simulink model "newnewPMSG"  (R2025b)
settings: Solver=VariableStepAuto  StartTime=0.0  StopTime=0.5  RelTol=1e-3
libraries: fl_lib x30, nesl_utility x19, ee_lib x8, simulink x7, slpidlib x6, eeTransforms x4, eePowerMeasurement x1, eeSinusoidalMeasurementV2 x1, mcbeeMathTransformLib x1
(part 1 of 2)
settings Model: SimulationMode=accelerator  Creator=zxd3816  LastModifiedBy=agarcian
settings SolverCC: AlgebraicLoopSolver=TrustRegion
settings DebuggingCC: UnconnectedInputMsg=warning  UnconnectedOutputMsg=warning  UnconnectedLineMsg=warning
settings ModelReferenceCC: EnableRefExpFcnMdlSchedulingChecks=on
settings RTWCC: GPUComputeCapability=3.5  DLArmComputeVersion=19.05

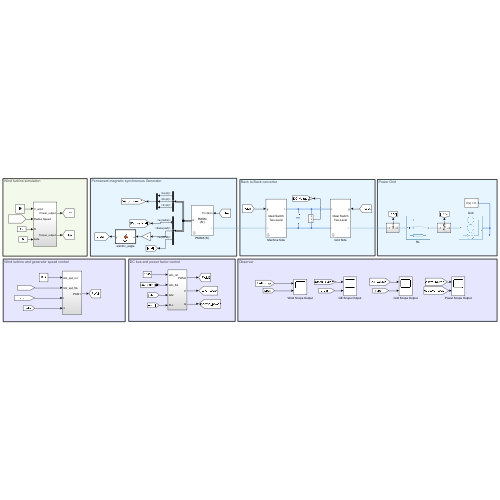
[thumbnail: Simulink's stored preview of the top-level diagram]
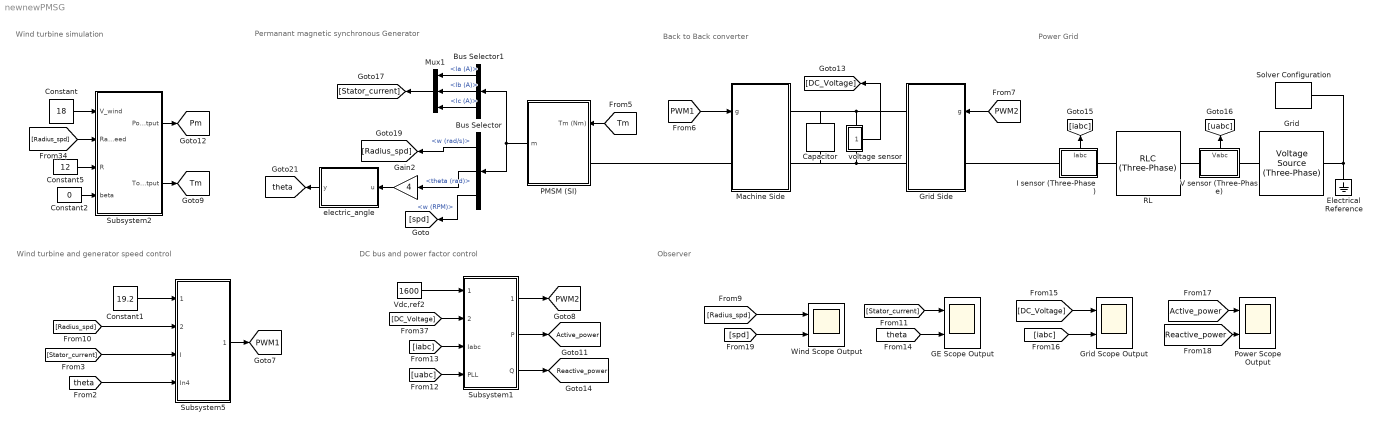
== system newnewPMSG ==
  note: DC bus and power factor control
  note: Wind turbine and generator speed control
  note: Wind turbine simulation
  note: Permanant magnetic synchronous Generator
  note: Power Grid
  note: Back to Back converter
  note: Observer
  Bus Selector : BusSelector  OutputSignals=w (rad/s),theta (rad),w (RPM)
  Bus Selector1 : BusSelector  OutputSignals=Ia (A),Ib (A),Ic (A)
  Capacitor : fl_lib/Electrical/Electrical Elements/Capacitor  c=5000e-5 F  r=0 Ohm  g=0 1/Ohm  i_specify=off  i_priority=None  i=0 A  i_nominal_specify=off  i_nominal_value=1  i_nominal_unit=A  v_specify=off  v_priority=None  v=0 V  v_nominal_specify=off  v_nominal_value=1  v_nominal_unit=V  vc_specify=on  vc_priority=High  vc=1600 V  vc_nominal_specify=off  vc_nominal_value=1  vc_nominal_unit=V
  Constant : Constant  Value=18
  Constant1 : Constant  Value=19.2
  Constant2 : Constant  Value=0
  Constant5 : Constant  Value=12
  Electrical Reference : fl_lib/Electrical/Electrical Elements/Electrical Reference
  GE Scope Output : Scope  NumInputPorts=2
      settings: ActiveDisplayYMinimum=-1886.54614  ActiveDisplayYMaximum=1887.1481  DataLoggingDecimation=10  DataLoggingVariableName=GE
  Gain2 : Gain  Gain=4
  Grid : ee_lib/Sources/Voltage Source (Three-Phase)  vline_rms=400*sqrt(3) V  shift=0 deg  freq=60 Hz  impedance_option=0  SShortCircuit=1e6 A*V  XR=15  R=0.01 Ohm  L=3.97e-4 H  harmonic_option=0  harmonic_orders=[5, 7, 11, 13]  harmonic_ratios=[.1, .1, .1, .1]  G_parasitic=0 1/Ohm  I_specify=off  I_priority=None  I=[0, 0, 0] A  I_nominal_specify=off  I_nominal_value=1  I_nominal_unit=A
  Grid Scope Output : Scope  NumInputPorts=2
      settings: ActiveDisplayYMinimum=1597.69606  ActiveDisplayYMaximum=1613.06273  DataLoggingDecimation=10  DataLoggingVariableName=Grid
  Grid Side : Subsystem  mask{Vf=1e-3, Ron=1e-3, Goff=1e-5, run_time=off}
      mask prompts: Vf "Forward Voltage (Vf)"; Ron "On Resistance (Ohm)"; Goff "Off Conductance (1/Ohm)"; run_time "Set parameters to run-time (model does not recompile if parameters change value)"
      mask Callback run_time:
      | run_time = get_param(gcb,'run_time');
      | 
      | path_converter = [gcb,'/converter'];
      | 
      | switch run_time
      |     case 'off'
      |         pcr = 'compiletime';
      |     case 'on'
      |         pcr = 'runtime';
      | end
      | 
      | set_param(path_converter,'Ron_conf',pcr)
      | set_param(path_converter,'Goff_conf',pcr)
      | set_param(path_converter,'Vf_conf',pcr)
      mask DialogControl DescGroupVar Prompt: Two-Level Converter
      mask Display: disp('Ideal Switch\nTwo-Level')
  I sensor (Three-Phase) : Subsystem
      settings: PortSchema="{\"entries\":[{\"content\":{\"sides\":[{\"content\":{\"connectorIds\":[\"LConn1\"]},\"type\":\"ConnectorPlacement.EquallySpacedRectSide\",\"uuid\":\"66880061-d275-464c-ab2c-563a1dd2cd8b\"},{\"content\":{\"connectorIds\":[\"RConn1\"],\"side\":\"RIGHT\"},\"type\":\"ConnectorPlacement.EquallySpacedRectSide\",\"uuid\":\"61b04713-3835-4ea6-b554-2bb2ace28c8c\"},{\"content\":{\"connectorIds\":[\"Out1\"],\"side\":\"TOP\"},\"type\":\"ConnectorPlacement.EquallySpacedRectSide\",\"uuid\":\"be795a7c-014c-44ea-ab59-513af0394dbb\"}]},\"type\":\"ConnectorPlacement.EquallySpacedConnector\",\"uuid\":\"739e21ea-20b0-4a9e-9950-77186c3d44aa\"}],\"packageUris\":[\"http://schema.mathworks.com/mf0/Connector/R2020b\"],\"version\":\"1.0\"}"
  Machine Side : Subsystem  mask{Vf=1e-3, Ron=1e-3, Goff=1e-5, run_time=off}
      mask prompts: Vf "Forward Voltage (Vf)"; Ron "On Resistance (Ohm)"; Goff "Off Conductance (1/Ohm)"; run_time "Set parameters to run-time (model does not recompile if parameters change value)"
      mask Callback run_time:
      | run_time = get_param(gcb,'run_time');
      | 
      | path_converter = [gcb,'/converter'];
      | 
      | switch run_time
      |     case 'off'
      |         pcr = 'compiletime';
      |     case 'on'
      |         pcr = 'runtime';
      | end
      | 
      | set_param(path_converter,'Ron_conf',pcr)
      | set_param(path_converter,'Goff_conf',pcr)
      | set_param(path_converter,'Vf_conf',pcr)
      mask DialogControl DescGroupVar Prompt: Two-Level Converter
      mask Display: disp('Ideal Switch\nTwo-Level')
  Mux1 : Mux  Inputs=3
  PMSM (SI) : Subsystem  mask{p=4, flux_linkage=1, Ld=0.001, Lq=0.001, Rs=0.005, J=0.5, D=0}
      mask prompts: p "pole pairs"; flux_linkage "Flux linkage (Wb)"; Ld "Stator d-axis inductance (H)"; Lq "Stator q-axis inductance (H)"; Rs "Stator resistance per phase (Ohm)"; J "Rotor inertia (kg*m^2)"; D "Rotor damping (N*m*s/rad)"
      mask DialogControl DescGroupVar Prompt: PMSM (SI)
      mask Display: disp('PMSM\n(SI)')
  Power Scope Output : Scope  NumInputPorts=2
      settings: ActiveDisplayYMinimum=-41950.10673  ActiveDisplayYMaximum=152400.48726  DataLoggingDecimation=10  DataLoggingVariableName=power
  RL : ee_lib/Passive/RLC Assemblies/RLC (Three-Phase)  port_option=ee.enum.threePhasePort.composite  component_structure=ee.enum.rlc.structure.SeriesRL  R=3/8 Ohm  L=3e-3 H  C=1e-6 F  R_parasitic=0 Ohm  G_parasitic=0 1/Ohm  IL_specify=off  IL_priority=High  IL=[0, 0, 0] A  IL_nominal_specify=off  IL_nominal_value=1  IL_nominal_unit=A  VC_specify=off  VC_priority=High  VC=[0, 0, 0] V  VC_nominal_specify=off  VC_nominal_value=1  VC_nominal_unit=V
      settings: InternalSimscapePortConfiguration="{\"Bottom\":[],\"Left\":[{\"id\":\"N1\",\"label\":\"~1\",\"type\":\"foundation.electrical.three_phase\"}],\"Right\":[{\"id\":\"N2\",\"label\":\"~2\",\"type\":\"foundation.electrical.three_phase\"}],\"Top\":[]}"
  Solver Configuration : nesl_utility/Solver Configuration  PhysicalDomain=network_engine_domain  SubClassName=solver  LeftPortType=input  RightPortType=generic  Tones=[]  Harmonics=[]  SimulateNoise=off  Profile=off  UseLocalSampling=off  EnableSwitchedLinearOptims=on  FrequencyDomain=off  UseCCode=off  RelTol=0.001  AbsTol=0.001  MinStep=1e-09  ToWorkspace=off  RevertToSquareIcSolve=off  NumHomotopyIterations=100  PhasorMode=off  PhasorModeNumHarmonics=1  ConsistencySolver=NEWTON_XTOL_AFTER_FTOL  IndexReductionMethod=None  DoDC=off  ResidualTolerance=1e-09  ConsistencyTolSource=GLOBAL  ConsistencyAbsTol=0.001  ConsistencyRelTol=0.001  ConsistencyTolFactor=0.001  UseLocalSolver=on  LocalSolverChoice=NE_PARTITIONING_ADVANCER  ResolveIndetEquations=off  FunctionEvalNumThread=1  LocalSolverSampleTime=5e-6  DoFixedCost=off  MaxNonlinIter=1  MaxModeIter=2  ComputeImpulses=off  ImpulseIterations=2  LinearAlgebra=auto  LinearAlgebraNumThread=0  EquationFormulation=NE_TIME_EF  DelaysMemoryBudget=1024  AutomaticFiltering=off  FilteringTimeConstant=0.001  PartitionStorageMethod=AS_NEEDED  PartitionMemoryBudget=1024  PartitionMethod=ROBUST  MultibodyUseLocalSolver=off  MultibodyLocalSolverChoice=ODE1  MultibodyLocalSolverSampleTime=0.001
  Subsystem1 : Subsystem
  Subsystem2 : Subsystem
  Subsystem5 : Subsystem
  V sensor (Three-Phase) : Subsystem
      settings: PortSchema="{\"entries\":[{\"content\":{\"sides\":[{\"content\":{\"connectorIds\":[\"LConn1\"]},\"type\":\"ConnectorPlacement.EquallySpacedRectSide\",\"uuid\":\"66880061-d275-464c-ab2c-563a1dd2cd8b\"},{\"content\":{\"connectorIds\":[\"RConn1\"],\"side\":\"RIGHT\"},\"type\":\"ConnectorPlacement.EquallySpacedRectSide\",\"uuid\":\"61b04713-3835-4ea6-b554-2bb2ace28c8c\"},{\"content\":{\"connectorIds\":[\"Out1\"],\"side\":\"TOP\"},\"type\":\"ConnectorPlacement.EquallySpacedRectSide\",\"uuid\":\"be795a7c-014c-44ea-ab59-513af0394dbb\"}]},\"type\":\"ConnectorPlacement.EquallySpacedConnector\",\"uuid\":\"739e21ea-20b0-4a9e-9950-77186c3d44aa\"}],\"packageUris\":[\"http://schema.mathworks.com/mf0/Connector/R2020b\"],\"version\":\"1.0\"}"
  Vdc,ref2 : Constant  Value=1600
  Wind Scope Output : Scope  NumInputPorts=2
      settings: ActiveDisplayYMinimum=-2.5199526294188392  ActiveDisplayYMaximum=22.679573664769556  DataLoggingDecimation=10  DataLoggingVariableName=wind
  electric_angle : MATLAB Function  TreatAsAtomicUnit=on
  voltage sensor : Subsystem
      settings: PortSchema="{\"entries\":[{\"content\":{\"sides\":[{\"content\":{},\"type\":\"ConnectorPlacement.EquallySpacedRectSide\",\"uuid\":\"799648ba-196f-427a-9565-f64fffdae700\"},{\"content\":{\"connectorIds\":[\"Out1\"],\"side\":\"RIGHT\"},\"type\":\"ConnectorPlacement.EquallySpacedRectSide\",\"uuid\":\"662de5d5-c2ef-406c-9235-94a35f9d89fb\"},{\"content\":{\"connectorIds\":[\"LConn1\"],\"side\":\"TOP\"},\"type\":\"ConnectorPlacement.EquallySpacedRectSide\",\"uuid\":\"67dc8fec-98bd-426f-bbe6-5723f2587b12\"},{\"content\":{\"connectorIds\":[\"RConn1\"],\"side\":\"BOTTOM\"},\"type\":\"ConnectorPlacement.EquallySpacedRectSide\",\"uuid\":\"7e3d7354-1ab6-44d8-9b44-c988118d052c\"}]},\"type\":\"ConnectorPlacement.EquallySpacedConnector\",\"uuid\":\"3e33dbb3-529a-4788-9727-18d62c402281\"}],\"packageUris\":[\"http://schema.mathworks.com/mf0/Connector/R2020b\"],\"version\":\"1.0\"}"
  tag scope: Active_power=global, PWM1=global, PWM2=global, Pm=global, Reactive_power=global, Tm=global, theta=global
  wires:
  [Radius_spd] -> Subsystem5/2(GE_spd_fbk)
  [Stator_current] -> Subsystem5/3(I)
  [theta] -> Subsystem5/4(In4)
  [iabc] -> Subsystem1/3(Iabc)
  [DC_Voltage] -> Subsystem1/2(Udc_fbk)
  Constant2/1 -> Subsystem2/4(beta)
  Constant5/1 -> Subsystem2/3(R)
  Vdc,ref2/1 -> Subsystem1/1(Udc_ref)
  [uabc] -> Subsystem1/4(PLL)
  Subsystem5/1(PWM1) -> [PWM1]
  Subsystem1/1(PWM2) -> [PWM2]
  Subsystem2/2(Torque_output) -> [Tm]
  Subsystem2/1(Power_output) -> [Pm]
  [Stator_current] -> GE Scope Output/1
  [theta] -> GE Scope Output/2
  [DC_Voltage] -> Grid Scope Output/1
  [iabc] -> Grid Scope Output/2
  Subsystem1/2(P) -> [Active_power]
  Subsystem1/3(Q) -> [Reactive_power]
  [Active_power] -> Power Scope Output/1
  [Reactive_power] -> Power Scope Output/2
  [Radius_spd] -> Wind Scope Output/1
  [spd] -> Wind Scope Output/2
  Constant/1 -> Subsystem2/1(V_wind)
  [Radius_spd] -> Subsystem2/2(Radius Speed)
  Constant1/1 -> Subsystem5/1(GE_spd_ref)
  PMSM (SI)/1(m) -> Bus Selector/1, Bus Selector1/1
  Bus Selector1/3 -> Mux1/3  "<Ic (A)>"
  Bus Selector1/2 -> Mux1/2  "<Ib (A)>"
  Bus Selector1/1 -> Mux1/1  "<Ia (A)>"
  [Tm] -> PMSM (SI)/1(Tm (Nm))
  [PWM1] -> Machine Side/1(g)
  [PWM2] -> Grid Side/1(g)
  I sensor (Three-Phase)/1(Iabc) -> [iabc]
  V sensor (Three-Phase)/1(Vabc) -> [uabc]
  Mux1/1 -> [Stator_current]
  electric_angle/1(y) -> [theta]
  Gain2/1 -> electric_angle/1(u)
  voltage sensor/1(v) -> [DC_Voltage]
  Bus Selector/1 -> [Radius_spd]  "<w (rad/s)>"
  Bus Selector/2 -> Gain2/1  "<theta (rad)>"
  Bus Selector/3 -> [spd]  "<w (RPM)>"
  connections:
  PMSM (SI)/LConn1 -- Machine Side/LConn1
  voltage sensor/RConn1 -- Grid Side/RConn2 -- Machine Side/RConn2 -- Capacitor/RConn1
  voltage sensor/LConn1 -- Grid Side/RConn1 -- Machine Side/RConn1 -- Capacitor/LConn1
  Grid Side/LConn1 -- I sensor (Three-Phase)/LConn1
  RL/LConn1 -- I sensor (Three-Phase)/RConn1
  V sensor (Three-Phase)/LConn1 -- RL/RConn1
  Grid/RConn1 -- V sensor (Three-Phase)/RConn1
  Electrical Reference/LConn1 -- Solver Configuration/RConn1 -- Grid/LConn1

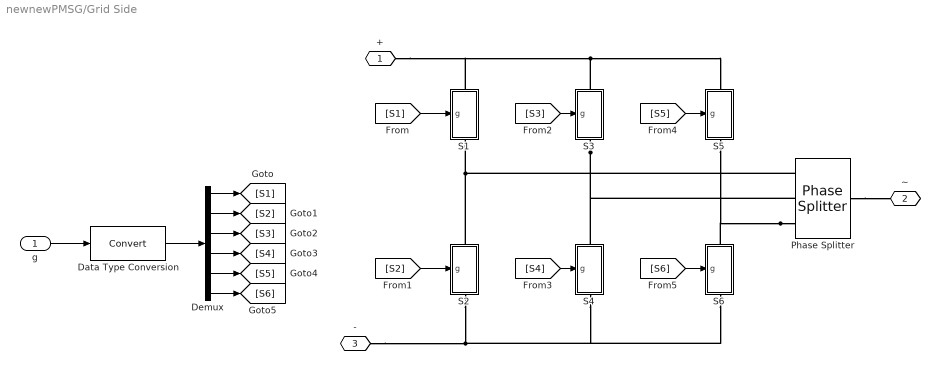
== system newnewPMSG/Grid Side ==
  g : Inport
  Data Type Conversion : DataTypeConversion  SaturateOnIntegerOverflow=off  RndMeth=Floor
  Demux : Demux  Outputs=6
  Phase Splitter : ee_lib/Connectors & References/Phase Splitter
  S1 : Subsystem
      settings: PortSchema="{\"entries\":[{\"content\":{\"sides\":[{\"content\":{\"connectorIds\":[\"In1\"]},\"type\":\"ConnectorPlacement.EquallySpacedRectSide\",\"uuid\":\"4868c43b-8f86-4e2f-a4da-367c2e17d6e4\"},{\"content\":{\"side\":\"RIGHT\"},\"type\":\"ConnectorPlacement.EquallySpacedRectSide\",\"uuid\":\"ebe9b5ec-833b-4a08-98e5-ff684cd7afcb\"},{\"content\":{\"connectorIds\":[\"LConn1\"],\"side\":\"TOP\"},\"type\":\"ConnectorPlacement.EquallySpacedRectSide\",\"uuid\":\"c72df866-8baa-41a8-9bb1-42a4a1fdee71\"},{\"content\":{\"connectorIds\":[\"RConn1\"],\"side\":\"BOTTOM\"},\"type\":\"ConnectorPlacement.EquallySpacedRectSide\",\"uuid\":\"3a9867c5-1563-48cb-a4f4-92deec85fd3d\"}]},\"type\":\"ConnectorPlacement.EquallySpacedConnector\",\"uuid\":\"206e0d7b-1d35-45e7-9c4c-8a6f9fe9dc79\"}],\"packageUris\":[\"http://schema.mathworks.com/mf0/Connector/R2020b\"],\"version\":\"1.0\"}"
  S2 : Subsystem
      settings: PortSchema="{\"entries\":[{\"content\":{\"sides\":[{\"content\":{\"connectorIds\":[\"In1\"]},\"type\":\"ConnectorPlacement.EquallySpacedRectSide\",\"uuid\":\"4868c43b-8f86-4e2f-a4da-367c2e17d6e4\"},{\"content\":{\"side\":\"RIGHT\"},\"type\":\"ConnectorPlacement.EquallySpacedRectSide\",\"uuid\":\"ebe9b5ec-833b-4a08-98e5-ff684cd7afcb\"},{\"content\":{\"connectorIds\":[\"LConn1\"],\"side\":\"TOP\"},\"type\":\"ConnectorPlacement.EquallySpacedRectSide\",\"uuid\":\"c72df866-8baa-41a8-9bb1-42a4a1fdee71\"},{\"content\":{\"connectorIds\":[\"RConn1\"],\"side\":\"BOTTOM\"},\"type\":\"ConnectorPlacement.EquallySpacedRectSide\",\"uuid\":\"3a9867c5-1563-48cb-a4f4-92deec85fd3d\"}]},\"type\":\"ConnectorPlacement.EquallySpacedConnector\",\"uuid\":\"206e0d7b-1d35-45e7-9c4c-8a6f9fe9dc79\"}],\"packageUris\":[\"http://schema.mathworks.com/mf0/Connector/R2020b\"],\"version\":\"1.0\"}"
  S3 : Subsystem
      settings: PortSchema="{\"entries\":[{\"content\":{\"sides\":[{\"content\":{\"connectorIds\":[\"In1\"]},\"type\":\"ConnectorPlacement.EquallySpacedRectSide\",\"uuid\":\"4868c43b-8f86-4e2f-a4da-367c2e17d6e4\"},{\"content\":{\"side\":\"RIGHT\"},\"type\":\"ConnectorPlacement.EquallySpacedRectSide\",\"uuid\":\"ebe9b5ec-833b-4a08-98e5-ff684cd7afcb\"},{\"content\":{\"connectorIds\":[\"LConn1\"],\"side\":\"TOP\"},\"type\":\"ConnectorPlacement.EquallySpacedRectSide\",\"uuid\":\"c72df866-8baa-41a8-9bb1-42a4a1fdee71\"},{\"content\":{\"connectorIds\":[\"RConn1\"],\"side\":\"BOTTOM\"},\"type\":\"ConnectorPlacement.EquallySpacedRectSide\",\"uuid\":\"3a9867c5-1563-48cb-a4f4-92deec85fd3d\"}]},\"type\":\"ConnectorPlacement.EquallySpacedConnector\",\"uuid\":\"206e0d7b-1d35-45e7-9c4c-8a6f9fe9dc79\"}],\"packageUris\":[\"http://schema.mathworks.com/mf0/Connector/R2020b\"],\"version\":\"1.0\"}"
  S4 : Subsystem
      settings: PortSchema="{\"entries\":[{\"content\":{\"sides\":[{\"content\":{\"connectorIds\":[\"In1\"]},\"type\":\"ConnectorPlacement.EquallySpacedRectSide\",\"uuid\":\"4868c43b-8f86-4e2f-a4da-367c2e17d6e4\"},{\"content\":{\"side\":\"RIGHT\"},\"type\":\"ConnectorPlacement.EquallySpacedRectSide\",\"uuid\":\"ebe9b5ec-833b-4a08-98e5-ff684cd7afcb\"},{\"content\":{\"connectorIds\":[\"LConn1\"],\"side\":\"TOP\"},\"type\":\"ConnectorPlacement.EquallySpacedRectSide\",\"uuid\":\"c72df866-8baa-41a8-9bb1-42a4a1fdee71\"},{\"content\":{\"connectorIds\":[\"RConn1\"],\"side\":\"BOTTOM\"},\"type\":\"ConnectorPlacement.EquallySpacedRectSide\",\"uuid\":\"3a9867c5-1563-48cb-a4f4-92deec85fd3d\"}]},\"type\":\"ConnectorPlacement.EquallySpacedConnector\",\"uuid\":\"206e0d7b-1d35-45e7-9c4c-8a6f9fe9dc79\"}],\"packageUris\":[\"http://schema.mathworks.com/mf0/Connector/R2020b\"],\"version\":\"1.0\"}"
  S5 : Subsystem
      settings: PortSchema="{\"entries\":[{\"content\":{\"sides\":[{\"content\":{\"connectorIds\":[\"In1\"]},\"type\":\"ConnectorPlacement.EquallySpacedRectSide\",\"uuid\":\"4868c43b-8f86-4e2f-a4da-367c2e17d6e4\"},{\"content\":{\"side\":\"RIGHT\"},\"type\":\"ConnectorPlacement.EquallySpacedRectSide\",\"uuid\":\"ebe9b5ec-833b-4a08-98e5-ff684cd7afcb\"},{\"content\":{\"connectorIds\":[\"LConn1\"],\"side\":\"TOP\"},\"type\":\"ConnectorPlacement.EquallySpacedRectSide\",\"uuid\":\"c72df866-8baa-41a8-9bb1-42a4a1fdee71\"},{\"content\":{\"connectorIds\":[\"RConn1\"],\"side\":\"BOTTOM\"},\"type\":\"ConnectorPlacement.EquallySpacedRectSide\",\"uuid\":\"3a9867c5-1563-48cb-a4f4-92deec85fd3d\"}]},\"type\":\"ConnectorPlacement.EquallySpacedConnector\",\"uuid\":\"206e0d7b-1d35-45e7-9c4c-8a6f9fe9dc79\"}],\"packageUris\":[\"http://schema.mathworks.com/mf0/Connector/R2020b\"],\"version\":\"1.0\"}"
  S6 : Subsystem
      settings: PortSchema="{\"entries\":[{\"content\":{\"sides\":[{\"content\":{\"connectorIds\":[\"In1\"]},\"type\":\"ConnectorPlacement.EquallySpacedRectSide\",\"uuid\":\"4868c43b-8f86-4e2f-a4da-367c2e17d6e4\"},{\"content\":{\"side\":\"RIGHT\"},\"type\":\"ConnectorPlacement.EquallySpacedRectSide\",\"uuid\":\"ebe9b5ec-833b-4a08-98e5-ff684cd7afcb\"},{\"content\":{\"connectorIds\":[\"LConn1\"],\"side\":\"TOP\"},\"type\":\"ConnectorPlacement.EquallySpacedRectSide\",\"uuid\":\"c72df866-8baa-41a8-9bb1-42a4a1fdee71\"},{\"content\":{\"connectorIds\":[\"RConn1\"],\"side\":\"BOTTOM\"},\"type\":\"ConnectorPlacement.EquallySpacedRectSide\",\"uuid\":\"3a9867c5-1563-48cb-a4f4-92deec85fd3d\"}]},\"type\":\"ConnectorPlacement.EquallySpacedConnector\",\"uuid\":\"206e0d7b-1d35-45e7-9c4c-8a6f9fe9dc79\"}],\"packageUris\":[\"http://schema.mathworks.com/mf0/Connector/R2020b\"],\"version\":\"1.0\"}"
  + : PMIOPort  Side=Right
  "~ " : PMIOPort  Port=2  Side=Left
  - : PMIOPort  Port=3  Side=Right
  wires:
  [S6] -> S6/1(g)
  [S4] -> S4/1(g)
  [S2] -> S2/1(g)
  [S1] -> S1/1(g)
  [S5] -> S5/1(g)
  [S3] -> S3/1(g)
  Demux/3 -> [S3]
  Demux/4 -> [S4]
  Demux/5 -> [S5]
  Demux/6 -> [S6]
  Demux/2 -> [S2]
  Demux/1 -> [S1]
  Data Type Conversion/1 -> Demux/1
  g/1 -> Data Type Conversion/1
  connections:
  S4/RConn1 -- S6/RConn1 -- -/RConn1 -- S2/RConn1
  S3/LConn1 -- S1/LConn1 -- +/RConn1 -- S5/LConn1
  Phase Splitter/RConn3 -- S5/RConn1 -- S6/LConn1
  S3/RConn1 -- Phase Splitter/RConn2 -- S4/LConn1
  S2/LConn1 -- S1/RConn1 -- Phase Splitter/RConn1
  Phase Splitter/LConn1 -- "~ "/RConn1

== system newnewPMSG/I sensor (Three-Phase) ==
  Current Sensor (Three-Phase) : ee_lib/Sensors & Transducers/Current Sensor (Three-Phase)
  PS-Simulink Converter1 : nesl_utility/PS-Simulink Converter  PhysicalDomain=network_engine_domain  SubClassName=ps_output  LeftPortType=input  RightPortType=output  PseudoPeriodic=off  Frequencies=[]  VectorFormat=inherit  Unit=inherit  AffineConversion=off
  ~1 : PMIOPort  Side=Left
  ~2 : PMIOPort  Port=2  Side=Right
  Iabc : Outport
  wires:
  PS-Simulink Converter1/1 -> Iabc/1
  connections:
  Current Sensor (Three-Phase)/RConn1 -- PS-Simulink Converter1/LConn1
  Current Sensor (Three-Phase)/LConn1 -- ~1/RConn1
  Current Sensor (Three-Phase)/RConn2 -- ~2/RConn1

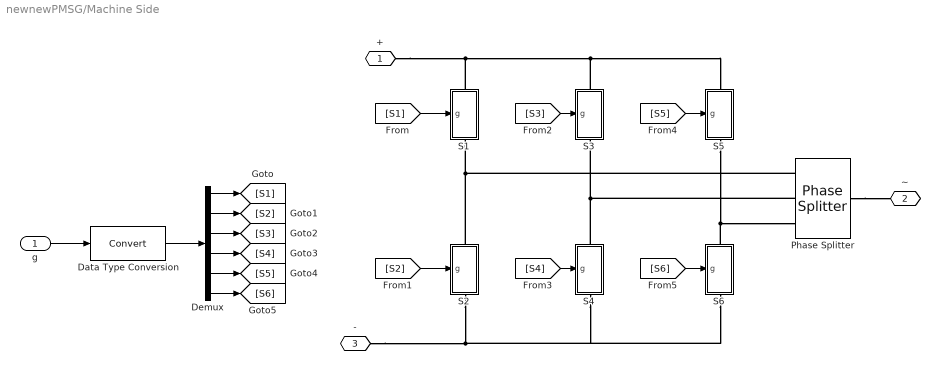
== system newnewPMSG/Machine Side ==
  g : Inport
  Data Type Conversion : DataTypeConversion  SaturateOnIntegerOverflow=off  RndMeth=Floor
  Demux : Demux  Outputs=6
  Phase Splitter : ee_lib/Connectors & References/Phase Splitter
  S1 : Subsystem
      settings: PortSchema="{\"entries\":[{\"content\":{\"sides\":[{\"content\":{\"connectorIds\":[\"In1\"]},\"type\":\"ConnectorPlacement.EquallySpacedRectSide\",\"uuid\":\"4868c43b-8f86-4e2f-a4da-367c2e17d6e4\"},{\"content\":{\"side\":\"RIGHT\"},\"type\":\"ConnectorPlacement.EquallySpacedRectSide\",\"uuid\":\"ebe9b5ec-833b-4a08-98e5-ff684cd7afcb\"},{\"content\":{\"connectorIds\":[\"LConn1\"],\"side\":\"TOP\"},\"type\":\"ConnectorPlacement.EquallySpacedRectSide\",\"uuid\":\"c72df866-8baa-41a8-9bb1-42a4a1fdee71\"},{\"content\":{\"connectorIds\":[\"RConn1\"],\"side\":\"BOTTOM\"},\"type\":\"ConnectorPlacement.EquallySpacedRectSide\",\"uuid\":\"3a9867c5-1563-48cb-a4f4-92deec85fd3d\"}]},\"type\":\"ConnectorPlacement.EquallySpacedConnector\",\"uuid\":\"206e0d7b-1d35-45e7-9c4c-8a6f9fe9dc79\"}],\"packageUris\":[\"http://schema.mathworks.com/mf0/Connector/R2020b\"],\"version\":\"1.0\"}"
  S2 : Subsystem
      settings: PortSchema="{\"entries\":[{\"content\":{\"sides\":[{\"content\":{\"connectorIds\":[\"In1\"]},\"type\":\"ConnectorPlacement.EquallySpacedRectSide\",\"uuid\":\"4868c43b-8f86-4e2f-a4da-367c2e17d6e4\"},{\"content\":{\"side\":\"RIGHT\"},\"type\":\"ConnectorPlacement.EquallySpacedRectSide\",\"uuid\":\"ebe9b5ec-833b-4a08-98e5-ff684cd7afcb\"},{\"content\":{\"connectorIds\":[\"LConn1\"],\"side\":\"TOP\"},\"type\":\"ConnectorPlacement.EquallySpacedRectSide\",\"uuid\":\"c72df866-8baa-41a8-9bb1-42a4a1fdee71\"},{\"content\":{\"connectorIds\":[\"RConn1\"],\"side\":\"BOTTOM\"},\"type\":\"ConnectorPlacement.EquallySpacedRectSide\",\"uuid\":\"3a9867c5-1563-48cb-a4f4-92deec85fd3d\"}]},\"type\":\"ConnectorPlacement.EquallySpacedConnector\",\"uuid\":\"206e0d7b-1d35-45e7-9c4c-8a6f9fe9dc79\"}],\"packageUris\":[\"http://schema.mathworks.com/mf0/Connector/R2020b\"],\"version\":\"1.0\"}"
  S3 : Subsystem
      settings: PortSchema="{\"entries\":[{\"content\":{\"sides\":[{\"content\":{\"connectorIds\":[\"In1\"]},\"type\":\"ConnectorPlacement.EquallySpacedRectSide\",\"uuid\":\"4868c43b-8f86-4e2f-a4da-367c2e17d6e4\"},{\"content\":{\"side\":\"RIGHT\"},\"type\":\"ConnectorPlacement.EquallySpacedRectSide\",\"uuid\":\"ebe9b5ec-833b-4a08-98e5-ff684cd7afcb\"},{\"content\":{\"connectorIds\":[\"LConn1\"],\"side\":\"TOP\"},\"type\":\"ConnectorPlacement.EquallySpacedRectSide\",\"uuid\":\"c72df866-8baa-41a8-9bb1-42a4a1fdee71\"},{\"content\":{\"connectorIds\":[\"RConn1\"],\"side\":\"BOTTOM\"},\"type\":\"ConnectorPlacement.EquallySpacedRectSide\",\"uuid\":\"3a9867c5-1563-48cb-a4f4-92deec85fd3d\"}]},\"type\":\"ConnectorPlacement.EquallySpacedConnector\",\"uuid\":\"206e0d7b-1d35-45e7-9c4c-8a6f9fe9dc79\"}],\"packageUris\":[\"http://schema.mathworks.com/mf0/Connector/R2020b\"],\"version\":\"1.0\"}"
  S4 : Subsystem
      settings: PortSchema="{\"entries\":[{\"content\":{\"sides\":[{\"content\":{\"connectorIds\":[\"In1\"]},\"type\":\"ConnectorPlacement.EquallySpacedRectSide\",\"uuid\":\"4868c43b-8f86-4e2f-a4da-367c2e17d6e4\"},{\"content\":{\"side\":\"RIGHT\"},\"type\":\"ConnectorPlacement.EquallySpacedRectSide\",\"uuid\":\"ebe9b5ec-833b-4a08-98e5-ff684cd7afcb\"},{\"content\":{\"connectorIds\":[\"LConn1\"],\"side\":\"TOP\"},\"type\":\"ConnectorPlacement.EquallySpacedRectSide\",\"uuid\":\"c72df866-8baa-41a8-9bb1-42a4a1fdee71\"},{\"content\":{\"connectorIds\":[\"RConn1\"],\"side\":\"BOTTOM\"},\"type\":\"ConnectorPlacement.EquallySpacedRectSide\",\"uuid\":\"3a9867c5-1563-48cb-a4f4-92deec85fd3d\"}]},\"type\":\"ConnectorPlacement.EquallySpacedConnector\",\"uuid\":\"206e0d7b-1d35-45e7-9c4c-8a6f9fe9dc79\"}],\"packageUris\":[\"http://schema.mathworks.com/mf0/Connector/R2020b\"],\"version\":\"1.0\"}"
  S5 : Subsystem
      settings: PortSchema="{\"entries\":[{\"content\":{\"sides\":[{\"content\":{\"connectorIds\":[\"In1\"]},\"type\":\"ConnectorPlacement.EquallySpacedRectSide\",\"uuid\":\"4868c43b-8f86-4e2f-a4da-367c2e17d6e4\"},{\"content\":{\"side\":\"RIGHT\"},\"type\":\"ConnectorPlacement.EquallySpacedRectSide\",\"uuid\":\"ebe9b5ec-833b-4a08-98e5-ff684cd7afcb\"},{\"content\":{\"connectorIds\":[\"LConn1\"],\"side\":\"TOP\"},\"type\":\"ConnectorPlacement.EquallySpacedRectSide\",\"uuid\":\"c72df866-8baa-41a8-9bb1-42a4a1fdee71\"},{\"content\":{\"connectorIds\":[\"RConn1\"],\"side\":\"BOTTOM\"},\"type\":\"ConnectorPlacement.EquallySpacedRectSide\",\"uuid\":\"3a9867c5-1563-48cb-a4f4-92deec85fd3d\"}]},\"type\":\"ConnectorPlacement.EquallySpacedConnector\",\"uuid\":\"206e0d7b-1d35-45e7-9c4c-8a6f9fe9dc79\"}],\"packageUris\":[\"http://schema.mathworks.com/mf0/Connector/R2020b\"],\"version\":\"1.0\"}"
  S6 : Subsystem
      settings: PortSchema="{\"entries\":[{\"content\":{\"sides\":[{\"content\":{\"connectorIds\":[\"In1\"]},\"type\":\"ConnectorPlacement.EquallySpacedRectSide\",\"uuid\":\"4868c43b-8f86-4e2f-a4da-367c2e17d6e4\"},{\"content\":{\"side\":\"RIGHT\"},\"type\":\"ConnectorPlacement.EquallySpacedRectSide\",\"uuid\":\"ebe9b5ec-833b-4a08-98e5-ff684cd7afcb\"},{\"content\":{\"connectorIds\":[\"LConn1\"],\"side\":\"TOP\"},\"type\":\"ConnectorPlacement.EquallySpacedRectSide\",\"uuid\":\"c72df866-8baa-41a8-9bb1-42a4a1fdee71\"},{\"content\":{\"connectorIds\":[\"RConn1\"],\"side\":\"BOTTOM\"},\"type\":\"ConnectorPlacement.EquallySpacedRectSide\",\"uuid\":\"3a9867c5-1563-48cb-a4f4-92deec85fd3d\"}]},\"type\":\"ConnectorPlacement.EquallySpacedConnector\",\"uuid\":\"206e0d7b-1d35-45e7-9c4c-8a6f9fe9dc79\"}],\"packageUris\":[\"http://schema.mathworks.com/mf0/Connector/R2020b\"],\"version\":\"1.0\"}"
  + : PMIOPort  Side=Right
  "~ " : PMIOPort  Port=2  Side=Left
  - : PMIOPort  Port=3  Side=Right
  wires:
  g/1 -> Data Type Conversion/1
  Data Type Conversion/1 -> Demux/1
  Demux/1 -> [S1]
  Demux/2 -> [S2]
  Demux/6 -> [S6]
  Demux/5 -> [S5]
  Demux/4 -> [S4]
  Demux/3 -> [S3]
  [S3] -> S3/1(g)
  [S5] -> S5/1(g)
  [S1] -> S1/1(g)
  [S2] -> S2/1(g)
  [S4] -> S4/1(g)
  [S6] -> S6/1(g)
  connections:
  Phase Splitter/LConn1 -- "~ "/RConn1
  Phase Splitter/RConn1 -- S2/LConn1 -- S1/RConn1
  Phase Splitter/RConn2 -- S4/LConn1 -- S3/RConn1
  S6/LConn1 -- S5/RConn1 -- Phase Splitter/RConn3
  +/RConn1 -- S3/LConn1 -- S5/LConn1 -- S1/LConn1
  -/RConn1 -- S6/RConn1 -- S4/RConn1 -- S2/RConn1

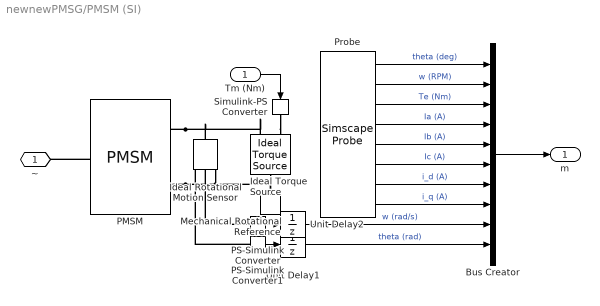
== system newnewPMSG/PMSM (SI) ==
  Tm (Nm) : Inport
  Bus Creator : BusCreator  Inputs=10
  Ideal Rotational Motion Sensor : fl_lib/Mechanical/Mechanical Sensors/Ideal Rotational Motion Sensor  reference=foundation.enum.MeasurementReference.difference  acceleration_port=false  velocity_port=true  position_port=true  wrap_angle=false  offset=0 rad
  Ideal Torque Source : fl_lib/Mechanical/Mechanical Sources/Ideal Torque Source
  Mechanical Rotational Reference : fl_lib/Mechanical/Rotational Elements/Mechanical Rotational Reference
  PMSM : ee_lib/Electromechanical/Permanent Magnet/PMSM  port_option=ee.enum.threePhasePort.composite  winding_type=ee.enum.electromech.statorconfiguration.wye  machine_param=ee.enum.pmsm.parameterization.constant  nPolePairs=p  pmflux_param=ee.enum.pmflux.fluxlinkage  pm_flux_linkage=flux_linkage Wb  torque_constant=0.18 N*m/A  back_emf_constant=0.18 V*s/rad  stator_param=ee.enum.statorparam.LdLqL0  Ld=Ld H  Lq=Lq H  idVec=[-200, 0, 200] A  iqVec=[-200, 0, 200] A  LdMatrix=0.0002 * ones(3, 3) H  LqMatrix=0.0002 * ones(3, 3) H  PmMatrix=0.1 * ones(3, 3) Wb  ktMatrix=0.18 * ones(3, 3) N*m/A  keMatrix=0.18 * ones(3, 3) V*s/rad  L0=0.00016 H  Ls=0.0002 H  Lm=-0.00002 H  Ms=0.00002 H  Rs=Rs Ohm  zero_sequence=ee.enum.park.zerosequence.exclude  axes_param=ee.enum.rotorangle.daxis  loss_param=ee.enum.ironloss.none  losses_oc=[0, 0, 0] W  losses_sc=[0, 0, 0] W  f_losses=60 Hz  Isc_losses=95 A  J=J kg*m^2  lam=D N*m*s/rad  i_d_specify=off  i_d_priority=None  i_d=0 A  i_d_nominal_specify=off  i_d_nominal_value=1  i_d_nominal_unit=A  i_q_specify=off  i_q_priority=None  i_q=0 A  i_q_nominal_specify=off  i_q_nominal_value=1  i_q_nominal_unit=A  torque_specify=off  torque_priority=None  torque=0 N*m  torque_nominal_specify=off  torque_nominal_value=1  torque_nominal_unit=N*m  angular_velocity_specify=off  angular_velocity_priority=High  angular_velocity=0 rpm  angular_velocity_nominal_specify=off  angular_velocity_nominal_value=1  angular_velocity_nominal_unit=rpm  angular_position_specify=off  angular_position_priority=High  angular_position=0 deg  angular_position_nominal_specify=off  angular_position_nominal_value=1  angular_position_nominal_unit=deg  alpha=3.93e-3 1/K  alpha_flux=-0.001 1/K  Tmeas=298.15 K  stator_thermal_mass=100 J/K  rotor_thermal_mass=200 J/K  Rm_percent_rotor=90  Rd_percent_rotor=30  temperatureA_specify=off  temperatureA_priority=High  temperatureA=25 degC  temperatureA_nominal_specify=off  temperatureA_nominal_value=1  temperatureA_nominal_unit=degC  temperatureB_specify=off  temperatureB_priority=High  temperatureB=25 degC  temperatureB_nominal_specify=off  temperatureB_nominal_value=1  temperatureB_nominal_unit=degC  temperatureC_specify=off  temperatureC_priority=High  temperatureC=25 degC  temperatureC_nominal_specify=off  temperatureC_nominal_value=1  temperatureC_nominal_unit=degC  temperatureR_specify=off  temperatureR_priority=High  temperatureR=25 degC  temperatureR_nominal_specify=off  temperatureR_nominal_value=1  temperatureR_nominal_unit=degC
      settings: InternalSimscapePortConfiguration="{\"Bottom\":[],\"Left\":[{\"id\":\"N\",\"label\":\"~\",\"type\":\"foundation.electrical.three_phase\"}],\"Right\":[{\"id\":\"R\",\"label\":\"R\",\"type\":\"foundation.mechanical.rotational.rotational\"},{\"id\":\"C\",\"label\":\"C\",\"type\":\"foundation.mechanical.rotational.rotational\"}],\"Top\":[]}"
  PS-Simulink Converter : nesl_utility/PS-Simulink Converter  PhysicalDomain=network_engine_domain  SubClassName=ps_output  LeftPortType=input  RightPortType=output  PseudoPeriodic=off  Frequencies=[]  VectorFormat=inherit  Unit=rad/s  AffineConversion=off
  PS-Simulink Converter1 : nesl_utility/PS-Simulink Converter  PhysicalDomain=network_engine_domain  SubClassName=ps_output  LeftPortType=input  RightPortType=output  PseudoPeriodic=off  Frequencies=[]  VectorFormat=inherit  Unit=rad  AffineConversion=off
  Probe : SimscapeProbe  BoundBlock=1156  Variables="{\"angular_position\":{\"Probing\":\"ON\"},\"angular_velocity\":{\"Probing\":\"ON\"},\"electrical_torque\":{\"Probing\":\"ON\"},\"i_a\":{\"Probing\":\"ON\"},\"i_b\":{\"Probing\":\"ON\"},\"i_c\":{\"Probing\":\"ON\"},\"i_d\":{\"Probing\":\"ON\"},\"i_q\":{\"Probing\":\"ON\"}}"
  Simulink-PS Converter : nesl_utility/Simulink-PS Converter  PhysicalDomain=network_engine_domain  SubClassName=ps_input  LeftPortType=input  RightPortType=output  PseudoPeriodic=off  Frequencies=[]  NoiseDistribution=none  NoiseParameters=[]  Unit=N*m  AffineConversion=off  FilteringAndDerivatives=provide  SimscapeFilterOrder=1  InputFilterTimeConstant=0.001  UdotUserProvided=0
  Unit Delay1 : UnitDelay  SampleTime=-1  HasFrameUpgradeWarning=on
  Unit Delay2 : UnitDelay  SampleTime=-1  HasFrameUpgradeWarning=on
  ~ : PMIOPort  Side=Left
  m : Outport
  wires:
  Bus Creator/1 -> m/1
  Probe/2 -> Bus Creator/2  "w (RPM)"
  Probe/3 -> Bus Creator/3  "Te (Nm)"
  Probe/1 -> Bus Creator/1  "theta (deg)"
  Tm (Nm)/1 -> Simulink-PS Converter/1
  PS-Simulink Converter1/1 -> Unit Delay1/1
  PS-Simulink Converter/1 -> Unit Delay2/1
  Probe/8 -> Bus Creator/8  "i_q (A)"
  Probe/7 -> Bus Creator/7  "i_d (A)"
  Probe/4 -> Bus Creator/4  "Ia (A)"
  Probe/5 -> Bus Creator/5  "Ib (A)"
  Probe/6 -> Bus Creator/6  "Ic (A)"
  Unit Delay1/1 -> Bus Creator/10  "theta (rad)"
  Unit Delay2/1 -> Bus Creator/9  "w (rad/s)"
  connections:
  PS-Simulink Converter1/LConn1 -- Ideal Rotational Motion Sensor/RConn3
  PS-Simulink Converter/LConn1 -- Ideal Rotational Motion Sensor/RConn2
  PMSM/RConn1 -- Ideal Rotational Motion Sensor/LConn1 -- Ideal Torque Source/RConn2
  Simulink-PS Converter/RConn1 -- Ideal Torque Source/RConn1
  PMSM/RConn2 -- Ideal Rotational Motion Sensor/RConn1 -- Ideal Torque Source/LConn1 -- Mechanical Rotational Reference/LConn1
  PMSM/LConn1 -- ~/RConn1

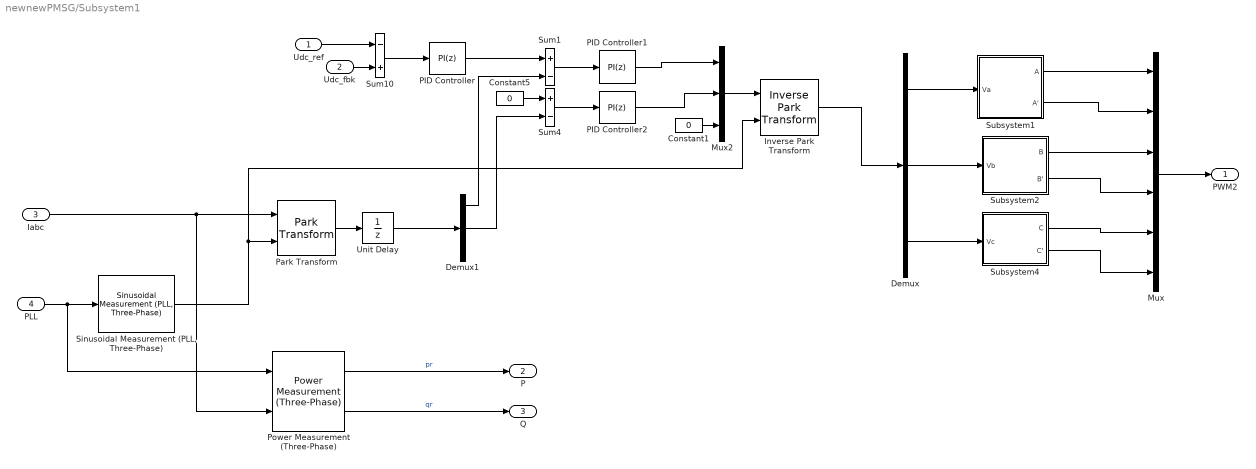
== system newnewPMSG/Subsystem1 ==
  Udc_ref : Inport
  Udc_fbk : Inport  Port=2
  Iabc : Inport  Port=3
  PLL : Inport  Port=4
  Constant1 : Constant  Value=0
  Constant5 : Constant  Value=0
  Demux : Demux  Outputs=3
  Demux1 : Demux  Outputs=3
  Inverse Park Transform : eeTransforms/Inverse Park Transform  AxisAlignment=Q-axis  PowerInvariant=off
      settings: LibrarySourceBlock=|
      | ee_sl_lib/Mathematical
      | Transforms/Inverse
      | Park Transform
  Mux : Mux  Inputs=6
  Mux2 : Mux  Inputs=3
  PID Controller : slpidlib/PID Controller  Controller=PI  Form=Parallel  TimeDomain=Discrete-time  UseExternalTs=off  SampleTime=-1  IntegratorMethod=Forward Euler  FilterMethod=Forward Euler  ControllerParametersSource=internal  P=1  I=100  UseKiTs=off  D=0  UseExternalDerivativeSource=off  N=100  UseFilter=on  TunerSelectOption=Transfer Function Based (PID Tuner App)  InitialConditionSource=internal  InitialConditionForIntegrator=0  InitialConditionForFilter=0  DifferentiatorICPrevScaledInput=0  ExternalReset=none  TrackingMode=off  Kt=1  LimitOutput=on  SatLimitsSource=internal  UpperSaturationLimit=500  LowerSaturationLimit=-500  LinearizeAsGain=on  AntiWindupMode=none  Kb=1  LimitIntegrator=off  UpperIntegratorSaturationLimit=inf  LowerIntegratorSaturationLimit=-inf  POutMin=[]  POutMax=[]  IOutMin=[]  IOutMax=[]  DOutMin=[]  DOutMax=[]  NOutMin=[]  NOutMax=[]  SumOutMin=[]  SumOutMax=[]  SaturationOutMin=[]  SaturationOutMax=[]  PParamMin=[]  PParamMax=[]  IParamMin=[]  IParamMax=[]  DParamMin=[]  DParamMax=[]  NParamMin=[]  NParamMax=[]  KbParamMin=[]  KbParamMax=[]  KtParamMin=[]  KtParamMax=[]  KbOutMin=[]  KbOutMax=[]  KtOutMin=[]  KtOutMax=[]  IntegratorOutMin=[]  IntegratorOutMax=[]  FilterOutMin=[]  FilterOutMax=[]  SumI1OutMin=[]  SumI1OutMax=[]  SumI2OutMin=[]  SumI2OutMax=[]  SumI3OutMin=[]  SumI3OutMax=[]  SumI4OutMin=[]  SumI4OutMax=[]  SumDOutMin=[]  SumDOutMax=[]  DifferentiatorOutMin=[]  DifferentiatorOutMax=[]  FilterDiffOutCoefMin=[]  FilterDiffOutCoefMax=[]  ReciprocalOutMin=[]  ReciprocalOutMax=[]  SumDenOutMin=[]  SumDenOutMax=[]  SumNumOutMin=[]  SumNumOutMax=[]  DivideOutMin=[]  DivideOutMax=[]  UdiffTsProdOutMin=[]  UdiffTsProdOutMax=[]  NTsProdOutMin=[]  NTsProdOutMax=[]  UintegralTsProdOutMin=[]  UintegralTsProdOutMax=[]  UngainTsProdOutMin=[]  UngainTsProdOutMax=[]  ClampingZeroOutDataTypeStr=Inherit: Inherit via back propagation  ClampingZeroOutMin=[]  ClampingZeroOutMax=[]  FilterDenConstantOutDataTypeStr=Inherit: Inherit via back propagation  FilterDenConstantOutMin=[]  FilterDenConstantOutMax=[]  PCopyOutDataTypeStr=Inherit: Inherit via back propagation  PCopyOutMin=[]  PCopyOutMax=[]  NCopyOutDataTypeStr=Inherit: Inherit via back propagation  NCopyOutMin=[]  NCopyOutMax=[]  IntegratorContinuousStateAttributes=''  IntegratorStateMustResolveToSignalObject=off  IntegratorRTWStateStorageClass=Auto  FilterContinuousStateAttributes=''  FilterStateMustResolveToSignalObject=off  FilterRTWStateStorageClass=Auto  ParallelPVariant=InternalParameters  IdealPVariant=Disabled  IVariant=InternalParameters  DVariant=Disabled  IntegratorVariant=Discrete  SatVariant=Enabled  AWVariant=Passthrough  PCopyVariant=Disabled  TRVariant=Disabled  FdbkBlocksVariant=Forward  IdealPFdbkVariant=Disabled  SatFdbkVariant=Disabled  DerivativeFilterVariant=Disabled  NVariant=Disabled  NCopyVariant=Disabled_SignalSpec  FilterICVariant=Disabled  IntegratorICVariant=InternalICs  ExternalResetVariant=Disabled  TRSumVariant=Passthrough  SumFdbkVariant=Disabled  SumVariant=Sum_PI  TsampFilterVariant=InternalTs  TsampNgainVariant=Passthrough  TsampIntegralVariant=Disabled_SignalSpec  ExternalSaturationOutDataTypeStr=Inherit: Same as second input  DerivativeSourceVariant=Disabled  PreIntVariant=InternalPreInt
  PID Controller1 : slpidlib/PID Controller  Controller=PI  Form=Parallel  TimeDomain=Discrete-time  UseExternalTs=off  SampleTime=-1  IntegratorMethod=Forward Euler  FilterMethod=Forward Euler  ControllerParametersSource=internal  P=0.16  I=20  UseKiTs=off  D=0  UseExternalDerivativeSource=off  N=100  UseFilter=on  TunerSelectOption=Transfer Function Based (PID Tuner App)  InitialConditionSource=internal  InitialConditionForIntegrator=0  InitialConditionForFilter=0  DifferentiatorICPrevScaledInput=0  ExternalReset=none  TrackingMode=off  Kt=1  LimitOutput=on  SatLimitsSource=internal  UpperSaturationLimit=6  LowerSaturationLimit=-6  LinearizeAsGain=on  AntiWindupMode=none  Kb=1  LimitIntegrator=off  UpperIntegratorSaturationLimit=inf  LowerIntegratorSaturationLimit=-inf  POutMin=[]  POutMax=[]  IOutMin=[]  IOutMax=[]  DOutMin=[]  DOutMax=[]  NOutMin=[]  NOutMax=[]  SumOutMin=[]  SumOutMax=[]  SaturationOutMin=[]  SaturationOutMax=[]  PParamMin=[]  PParamMax=[]  IParamMin=[]  IParamMax=[]  DParamMin=[]  DParamMax=[]  NParamMin=[]  NParamMax=[]  KbParamMin=[]  KbParamMax=[]  KtParamMin=[]  KtParamMax=[]  KbOutMin=[]  KbOutMax=[]  KtOutMin=[]  KtOutMax=[]  IntegratorOutMin=[]  IntegratorOutMax=[]  FilterOutMin=[]  FilterOutMax=[]  SumI1OutMin=[]  SumI1OutMax=[]  SumI2OutMin=[]  SumI2OutMax=[]  SumI3OutMin=[]  SumI3OutMax=[]  SumI4OutMin=[]  SumI4OutMax=[]  SumDOutMin=[]  SumDOutMax=[]  DifferentiatorOutMin=[]  DifferentiatorOutMax=[]  FilterDiffOutCoefMin=[]  FilterDiffOutCoefMax=[]  ReciprocalOutMin=[]  ReciprocalOutMax=[]  SumDenOutMin=[]  SumDenOutMax=[]  SumNumOutMin=[]  SumNumOutMax=[]  DivideOutMin=[]  DivideOutMax=[]  UdiffTsProdOutMin=[]  UdiffTsProdOutMax=[]  NTsProdOutMin=[]  NTsProdOutMax=[]  UintegralTsProdOutMin=[]  UintegralTsProdOutMax=[]  UngainTsProdOutMin=[]  UngainTsProdOutMax=[]  ClampingZeroOutDataTypeStr=Inherit: Inherit via back propagation  ClampingZeroOutMin=[]  ClampingZeroOutMax=[]  FilterDenConstantOutDataTypeStr=Inherit: Inherit via back propagation  FilterDenConstantOutMin=[]  FilterDenConstantOutMax=[]  PCopyOutDataTypeStr=Inherit: Inherit via back propagation  PCopyOutMin=[]  PCopyOutMax=[]  NCopyOutDataTypeStr=Inherit: Inherit via back propagation  NCopyOutMin=[]  NCopyOutMax=[]  IntegratorContinuousStateAttributes=''  IntegratorStateMustResolveToSignalObject=off  IntegratorRTWStateStorageClass=Auto  FilterContinuousStateAttributes=''  FilterStateMustResolveToSignalObject=off  FilterRTWStateStorageClass=Auto  ParallelPVariant=InternalParameters  IdealPVariant=Disabled  IVariant=InternalParameters  DVariant=Disabled  IntegratorVariant=Discrete  SatVariant=Enabled  AWVariant=Passthrough  PCopyVariant=Disabled  TRVariant=Disabled  FdbkBlocksVariant=Forward  IdealPFdbkVariant=Disabled  SatFdbkVariant=Disabled  DerivativeFilterVariant=Disabled  NVariant=Disabled  NCopyVariant=Disabled_SignalSpec  FilterICVariant=Disabled  IntegratorICVariant=InternalICs  ExternalResetVariant=Disabled  TRSumVariant=Passthrough  SumFdbkVariant=Disabled  SumVariant=Sum_PI  TsampFilterVariant=InternalTs  TsampNgainVariant=Passthrough  TsampIntegralVariant=Disabled_SignalSpec  ExternalSaturationOutDataTypeStr=Inherit: Same as second input  DerivativeSourceVariant=Disabled  PreIntVariant=InternalPreInt
  PID Controller2 : slpidlib/PID Controller  Controller=PI  Form=Parallel  TimeDomain=Discrete-time  UseExternalTs=off  SampleTime=-1  IntegratorMethod=Forward Euler  FilterMethod=Forward Euler  ControllerParametersSource=internal  P=0.16  I=20  UseKiTs=off  D=0  UseExternalDerivativeSource=off  N=100  UseFilter=on  TunerSelectOption=Transfer Function Based (PID Tuner App)  InitialConditionSource=internal  InitialConditionForIntegrator=0  InitialConditionForFilter=0  DifferentiatorICPrevScaledInput=0  ExternalReset=none  TrackingMode=off  Kt=1  LimitOutput=on  SatLimitsSource=internal  UpperSaturationLimit=6  LowerSaturationLimit=-6  LinearizeAsGain=on  AntiWindupMode=none  Kb=1  LimitIntegrator=off  UpperIntegratorSaturationLimit=inf  LowerIntegratorSaturationLimit=-inf  POutMin=[]  POutMax=[]  IOutMin=[]  IOutMax=[]  DOutMin=[]  DOutMax=[]  NOutMin=[]  NOutMax=[]  SumOutMin=[]  SumOutMax=[]  SaturationOutMin=[]  SaturationOutMax=[]  PParamMin=[]  PParamMax=[]  IParamMin=[]  IParamMax=[]  DParamMin=[]  DParamMax=[]  NParamMin=[]  NParamMax=[]  KbParamMin=[]  KbParamMax=[]  KtParamMin=[]  KtParamMax=[]  KbOutMin=[]  KbOutMax=[]  KtOutMin=[]  KtOutMax=[]  IntegratorOutMin=[]  IntegratorOutMax=[]  FilterOutMin=[]  FilterOutMax=[]  SumI1OutMin=[]  SumI1OutMax=[]  SumI2OutMin=[]  SumI2OutMax=[]  SumI3OutMin=[]  SumI3OutMax=[]  SumI4OutMin=[]  SumI4OutMax=[]  SumDOutMin=[]  SumDOutMax=[]  DifferentiatorOutMin=[]  DifferentiatorOutMax=[]  FilterDiffOutCoefMin=[]  FilterDiffOutCoefMax=[]  ReciprocalOutMin=[]  ReciprocalOutMax=[]  SumDenOutMin=[]  SumDenOutMax=[]  SumNumOutMin=[]  SumNumOutMax=[]  DivideOutMin=[]  DivideOutMax=[]  UdiffTsProdOutMin=[]  UdiffTsProdOutMax=[]  NTsProdOutMin=[]  NTsProdOutMax=[]  UintegralTsProdOutMin=[]  UintegralTsProdOutMax=[]  UngainTsProdOutMin=[]  UngainTsProdOutMax=[]  ClampingZeroOutDataTypeStr=Inherit: Inherit via back propagation  ClampingZeroOutMin=[]  ClampingZeroOutMax=[]  FilterDenConstantOutDataTypeStr=Inherit: Inherit via back propagation  FilterDenConstantOutMin=[]  FilterDenConstantOutMax=[]  PCopyOutDataTypeStr=Inherit: Inherit via back propagation  PCopyOutMin=[]  PCopyOutMax=[]  NCopyOutDataTypeStr=Inherit: Inherit via back propagation  NCopyOutMin=[]  NCopyOutMax=[]  IntegratorContinuousStateAttributes=''  IntegratorStateMustResolveToSignalObject=off  IntegratorRTWStateStorageClass=Auto  FilterContinuousStateAttributes=''  FilterStateMustResolveToSignalObject=off  FilterRTWStateStorageClass=Auto  ParallelPVariant=InternalParameters  IdealPVariant=Disabled  IVariant=InternalParameters  DVariant=Disabled  IntegratorVariant=Discrete  SatVariant=Enabled  AWVariant=Passthrough  PCopyVariant=Disabled  TRVariant=Disabled  FdbkBlocksVariant=Forward  IdealPFdbkVariant=Disabled  SatFdbkVariant=Disabled  DerivativeFilterVariant=Disabled  NVariant=Disabled  NCopyVariant=Disabled_SignalSpec  FilterICVariant=Disabled  IntegratorICVariant=InternalICs  ExternalResetVariant=Disabled  TRSumVariant=Passthrough  SumFdbkVariant=Disabled  SumVariant=Sum_PI  TsampFilterVariant=InternalTs  TsampNgainVariant=Passthrough  TsampIntegralVariant=Disabled_SignalSpec  ExternalSaturationOutDataTypeStr=Inherit: Same as second input  DerivativeSourceVariant=Disabled  PreIntVariant=InternalPreInt
  Park Transform : eeTransforms/Park Transform  AxisAlignment=Q-axis  PowerInvariant=off
      settings: LibrarySourceBlock=|
      | ee_sl_lib/Mathematical
      | Transforms/Park Transform
  Power Measurement (Three-Phase) : eePowerMeasurement/Power Measurement (Three-Phase)  LabelModeActiveChoice=Discrete  F=60  K=1  Seq=Positive  Ts=5e-6
  "Sinusoidal Measurement (PLL, Three-Phase)" : eeSinusoidalMeasurementV2/Sinusoidal Measurement (PLL, Three-Phase)  InputFilter=on  InputNormalization=off  Kp_LF=0.2  Ki_LF=8  F0=60  Theta0=0  Ts=5e-6
      settings: LibrarySourceBlock=|
      | ee_sl_lib/Measurements/Sinusoidal Measurement
      | (PLL, Three-Phase)
  Subsystem1 : Subsystem
  Subsystem2 : Subsystem
  Subsystem4 : Subsystem
  Sum1 : Sum  Inputs=+-
  Sum10 : Sum  Inputs=-+
  Sum4 : Sum  Inputs=+-
  Unit Delay : UnitDelay  SampleTime=-1  HasFrameUpgradeWarning=on
  PWM2 : Outport
  P : Outport  Port=2  VectorParamsAs1DForOutWhenUnconnected=off
  Q : Outport  Port=3  VectorParamsAs1DForOutWhenUnconnected=off
  wires:
  Udc_fbk/1 -> Sum10/2
  Udc_ref/1 -> Sum10/1
  PID Controller/1 -> Sum1/1
  Sum10/1 -> PID Controller/1
  Iabc/1 -> Park Transform/1, Power Measurement (Three-Phase)/2
  Sum4/1 -> PID Controller2/1
  Sum1/1 -> PID Controller1/1
  PLL/1 -> Power Measurement (Three-Phase)/1, "Sinusoidal Measurement (PLL, Three-Phase)"/1
  Park Transform/1 -> Unit Delay/1
  Constant5/1 -> Sum4/1
  Demux1/1 -> Sum1/2
  Demux1/2 -> Sum4/2
  Constant1/1 -> Mux2/3
  PID Controller2/1 -> Mux2/2
  PID Controller1/1 -> Mux2/1
  Inverse Park Transform/1 -> Demux/1
  Demux/1 -> Subsystem1/1(Va)
  Demux/2 -> Subsystem2/1(Vb)
  Demux/3 -> Subsystem4/1(Vc)
  Subsystem1/1(A) -> Mux/1
  Subsystem1/2(A') -> Mux/2
  Subsystem2/1(B) -> Mux/3
  Subsystem2/2(B') -> Mux/4
  Subsystem4/1(C) -> Mux/5
  Subsystem4/2(C') -> Mux/6
  Mux2/1 -> Inverse Park Transform/1
  Mux/1 -> PWM2/1
  Unit Delay/1 -> Demux1/1
  "Sinusoidal Measurement (PLL, Three-Phase)"/2 -> Inverse Park Transform/2, Park Transform/2
  Power Measurement (Three-Phase)/1 -> P/1  "pr"
  Power Measurement (Three-Phase)/2 -> Q/1  "qr"

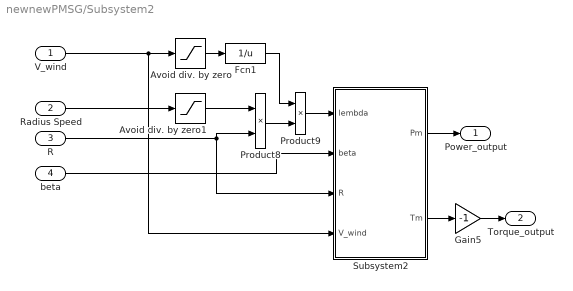
== system newnewPMSG/Subsystem2 ==
  V_wind : Inport
  Radius Speed : Inport  Port=2
  R : Inport  Port=3
  beta : Inport  Port=4
  Avoid div. by zero : Saturate  UpperLimit=inf  LowerLimit=eps
  Avoid div. by zero1 : Saturate  UpperLimit=inf  LowerLimit=eps
  Fcn1 : Fcn  Expr=1/u
  Gain5 : Gain  Gain=-1
  Product8 : Product  RndMeth=Zero
  Product9 : Product  RndMeth=Zero
  Subsystem2 : Subsystem
  Power_output : Outport  VectorParamsAs1DForOutWhenUnconnected=off
  Torque_output : Outport  Port=2  VectorParamsAs1DForOutWhenUnconnected=off
  wires:
  Product9/1 -> Subsystem2/1(lembda)
  V_wind/1 -> Subsystem2/4(V_wind), Avoid div. by zero/1
  Avoid div. by zero/1 -> Fcn1/1
  Product8/1 -> Product9/2
  Fcn1/1 -> Product9/1
  R/1 -> Product8/2, Subsystem2/3(R)
  Radius Speed/1 -> Avoid div. by zero1/1
  Subsystem2/2(Tm) -> Gain5/1
  beta/1 -> Subsystem2/2(beta)
  Gain5/1 -> Torque_output/1
  Subsystem2/1(Pm) -> Power_output/1
  Avoid div. by zero1/1 -> Product8/1
